simulink model "analyze"  (R2014a)
settings: Solver=FixedStepDiscrete  StartTime=0.0  StopTime=1  FixedStep=0.02  RelTol=1e-3
InitFcn:
  | Veh_Par_wxt
values from neighbouring files (symbols this model uses):
  ag_thr = 0.4*g    (= 3.924)    [Veh_Par_wxt.m]
  B = 2.25    [Veh_Par_wxt.m]
  bra_pre_em = 12    [Veh_Par_wxt.m]
  bra_pre_gz2 = 12/3    (= 4)    [Veh_Par_wxt.m]
  bra_pre_gz34 = 12/3    (= 4)    [Veh_Par_wxt.m]
  bra_pre_yd = 12/2    (= 6)    [Veh_Par_wxt.m]
  brakepre_dem_data = [0 1 2 3 4 5 6 7 8 9 10 11 12]    [Veh_Par_wxt.m]
  brakeTrq_dem_data = [0 218.198 436.396 654.594 872.792 1090.99 1309.188 1527.386 1745.584 1963.782 2181.98 2400.178 2618.376]    [Veh_Par_wxt.m]
  bratrq_max = 4*2618.376    (= 10473.504)    [Veh_Par_wxt.m]
  eff_tran = 0.75    [Veh_Par_wxt.m]
  G = Mass*g    (= 36297)    [Veh_Par_wxt.m]
  kd1 = 1    [Veh_Par_wxt.m]
  kd2 = 1    [Veh_Par_wxt.m]
  kd3 = 1    [Veh_Par_wxt.m]
  ki1 = 1    [Veh_Par_wxt.m]
  ki2 = 1    [Veh_Par_wxt.m]
  ki3 = 1    [Veh_Par_wxt.m]
  kp1 = 1    [Veh_Par_wxt.m]
  kp2 = 1    [Veh_Par_wxt.m]
  kp3 = 1    [Veh_Par_wxt.m]
  L = 3.12    [Veh_Par_wxt.m]
  premax = 12    [Veh_Par_wxt.m]
  Radius = 0.20    (= 0.2)    [Veh_Par_wxt.m]
  s_opt_yi_add = 0.05    [Veh_Par_wxt.m]
  s_opt_zhuan_add = 0.05    [Veh_Par_wxt.m]
  spd_map_mot = [0 100 200 300 360 400 500 600 700 800 900]*tras_ratio    [Veh_Par_wxt.m]
  spdmax = 900*tras_ratio    (= 5580)    [Veh_Par_wxt.m]
  speed_thr_park = 5/3.6/Radius*30/pi    (= 66.3145596216)    [Veh_Par_wxt.m]
  tras_ratio = 6.2    [Veh_Par_wxt.m]
  trq_map_mot = [1200 1200 1200 1200 1200 1080 864 720 617 540 480]/tras_ratio    [Veh_Par_wxt.m]
  trqmax = 80    [Veh_Par_wxt.m]
  v_thr1_b = 5    [Veh_Par_wxt.m]
  v_thr2_b = 20    [Veh_Par_wxt.m]
  v_thr_park = 5    [Veh_Par_wxt.m]
undefined symbols (not defined in the file or in its folder): DiscIntNeverNeededParam
libraries: simulink x231, ec5744lib x19
(part 3 of 16)

== system analyze/OutputSignalProcess/VCU_MCU2 ==
  M3Enable_in : Inport
  M3Mode_in : Inport  Port=2
  M3Drive_in : Inport  Port=3
  M3TorqueSet_in : Inport  Port=4
  M3SpeedLimit_in : Inport  Port=5
  M4Enable_in : Inport  Port=6
  M4Mode_in : Inport  Port=7
  M4Drive_in : Inport  Port=8
  M4TorqueSet_in : Inport  Port=9
  M4SpeedLimit_in : Inport  Port=10
  MCU2HeartBeat_in : Inport  Port=11
  Conv{1..8} (8 alike) : DataTypeConversion
  M3Drive : Subsystem
  M3Enable : Subsystem
  M3Mode : Subsystem
  M3SpeedLimit : Subsystem
  M3TorqueSet : Subsystem
  M4Drive : Subsystem
  M4Enable : Subsystem
  M4Mode : Subsystem
  M4SpeedLimit : Subsystem
  M4TorqueSet : Subsystem
  MCU2HeartBeat : Subsystem
  VCU_MCU2_DLC : Constant  Value=8  OutDataTypeStr=uint8
  VCU_MCU2_DLC_Out : Terminator
  VCU_MCU2_ID : Constant  Value=2348937218  OutDataTypeStr=single
  VCU_MCU2_ID_Out : Terminator
  VCU_MCU2_mux : Mux  Inputs=8
  or{1..8} (8 alike) : simulink/Logic and Bit Operations/Bitwise Operator  logicop=OR  UseBitMask=off  NumInputPorts=11  BitMask=bin2dec('11011001')  BitMaskRealWorld=Stored Integer
  output : Outport
  wires:
  VCU_MCU2_mux/1 -> output/1
  MCU2HeartBeat/1(output1) -> or1/1
  MCU2HeartBeat/2(output2) -> or2/1
  MCU2HeartBeat/3(output3) -> or3/1
  MCU2HeartBeat/4(output4) -> or4/1
  MCU2HeartBeat/5(output5) -> or5/1
  MCU2HeartBeat/6(output6) -> or6/1
  MCU2HeartBeat/7(output7) -> or7/1
  MCU2HeartBeat/8(output8) -> or8/1
  M4TorqueSet/1(output1) -> or1/2
  M4TorqueSet/2(output2) -> or2/2
  M4TorqueSet/3(output3) -> or3/2
  M4TorqueSet/4(output4) -> or4/2
  M4TorqueSet/5(output5) -> or5/2
  M4TorqueSet/6(output6) -> or6/2
  M4TorqueSet/7(output7) -> or7/2
  M4TorqueSet/8(output8) -> or8/2
  M4SpeedLimit/1(output1) -> or1/3
  M4SpeedLimit/2(output2) -> or2/3
  M4SpeedLimit/3(output3) -> or3/3
  M4SpeedLimit/4(output4) -> or4/3
  M4SpeedLimit/5(output5) -> or5/3
  M4SpeedLimit/6(output6) -> or6/3
  M4SpeedLimit/7(output7) -> or7/3
  M4SpeedLimit/8(output8) -> or8/3
  M4Mode/1(output1) -> or1/4
  M4Mode/2(output2) -> or2/4
  M4Mode/3(output3) -> or3/4
  M4Mode/4(output4) -> or4/4
  M4Mode/5(output5) -> or5/4
  M4Mode/6(output6) -> or6/4
  M4Mode/7(output7) -> or7/4
  M4Mode/8(output8) -> or8/4
  M4Enable/1(output1) -> or1/5
  M4Enable/2(output2) -> or2/5
  M4Enable/3(output3) -> or3/5
  M4Enable/4(output4) -> or4/5
  M4Enable/5(output5) -> or5/5
  M4Enable/6(output6) -> or6/5
  M4Enable/7(output7) -> or7/5
  M4Enable/8(output8) -> or8/5
  M4Drive/1(output1) -> or1/6
  M4Drive/2(output2) -> or2/6
  M4Drive/3(output3) -> or3/6
  M4Drive/4(output4) -> or4/6
  M4Drive/5(output5) -> or5/6
  M4Drive/6(output6) -> or6/6
  M4Drive/7(output7) -> or7/6
  M4Drive/8(output8) -> or8/6
  M3TorqueSet/1(output1) -> or1/7
  M3TorqueSet/2(output2) -> or2/7
  M3TorqueSet/3(output3) -> or3/7
  M3TorqueSet/4(output4) -> or4/7
  M3TorqueSet/5(output5) -> or5/7
  M3TorqueSet/6(output6) -> or6/7
  M3TorqueSet/7(output7) -> or7/7
  M3TorqueSet/8(output8) -> or8/7
  M3SpeedLimit/1(output1) -> or1/8
  M3SpeedLimit/2(output2) -> or2/8
  M3SpeedLimit/3(output3) -> or3/8
  M3SpeedLimit/4(output4) -> or4/8
  M3SpeedLimit/5(output5) -> or5/8
  M3SpeedLimit/6(output6) -> or6/8
  M3SpeedLimit/7(output7) -> or7/8
  M3SpeedLimit/8(output8) -> or8/8
  M3Mode/1(output1) -> or1/9
  M3Mode/2(output2) -> or2/9
  M3Mode/3(output3) -> or3/9
  M3Mode/4(output4) -> or4/9
  M3Mode/5(output5) -> or5/9
  M3Mode/6(output6) -> or6/9
  M3Mode/7(output7) -> or7/9
  M3Mode/8(output8) -> or8/9
  M3Enable/1(output1) -> or1/10
  M3Enable/2(output2) -> or2/10
  M3Enable/3(output3) -> or3/10
  M3Enable/4(output4) -> or4/10
  M3Enable/5(output5) -> or5/10
  M3Enable/6(output6) -> or6/10
  M3Enable/7(output7) -> or7/10
  M3Enable/8(output8) -> or8/10
  M3Drive/1(output1) -> or1/11
  M3Drive/2(output2) -> or2/11
  M3Drive/3(output3) -> or3/11
  M3Drive/4(output4) -> or4/11
  M3Drive/5(output5) -> or5/11
  M3Drive/6(output6) -> or6/11
  M3Drive/7(output7) -> or7/11
  M3Drive/8(output8) -> or8/11
  or1/1 -> Conv1/1
  Conv1/1 -> VCU_MCU2_mux/1
  or2/1 -> Conv2/1
  Conv2/1 -> VCU_MCU2_mux/2
  or3/1 -> Conv3/1
  Conv3/1 -> VCU_MCU2_mux/3
  or4/1 -> Conv4/1
  Conv4/1 -> VCU_MCU2_mux/4
  or5/1 -> Conv5/1
  Conv5/1 -> VCU_MCU2_mux/5
  or6/1 -> Conv6/1
  Conv6/1 -> VCU_MCU2_mux/6
  or7/1 -> Conv7/1
  Conv7/1 -> VCU_MCU2_mux/7
  or8/1 -> Conv8/1
  Conv8/1 -> VCU_MCU2_mux/8
  VCU_MCU2_ID/1 -> VCU_MCU2_ID_Out/1
  VCU_MCU2_DLC/1 -> VCU_MCU2_DLC_Out/1
  MCU2HeartBeat_in/1 -> MCU2HeartBeat/1(MCU2HeartBeat)
  M4TorqueSet_in/1 -> M4TorqueSet/1(M4TorqueSet)
  M4SpeedLimit_in/1 -> M4SpeedLimit/1(M4SpeedLimit)
  M4Mode_in/1 -> M4Mode/1(M4Mode)
  M4Enable_in/1 -> M4Enable/1(M4Enable)
  M4Drive_in/1 -> M4Drive/1(M4Drive)
  M3TorqueSet_in/1 -> M3TorqueSet/1(M3TorqueSet)
  M3SpeedLimit_in/1 -> M3SpeedLimit/1(M3SpeedLimit)
  M3Mode_in/1 -> M3Mode/1(M3Mode)
  M3Enable_in/1 -> M3Enable/1(M3Enable)
  M3Drive_in/1 -> M3Drive/1(M3Drive)

== matlab function analyze/MainControl/mode_control/forward/forward/Drive/驱动防滑控制TCS/转向TCS/右转/前后轮均滑转/HeartBeat1 ==
  data: life_pre input; life output
function life = fcn(life_pre)
%#codegen
life=life_pre+1;
if life>15
    life=0;
end
end

== matlab function analyze/MainControl/mode_control/forward/forward/Drive/驱动防滑控制TCS/转向TCS/右转/无滑转/HeartBeat1 ==
  data: life_pre input; life output
function life = fcn(life_pre)
%#codegen
life=life_pre+1;
if life>15
    life=0;
end
end

== matlab function analyze/MainControl/mode_control/forward/forward/Brake/MATLAB Function ==
  data: guzhang_lf input; gz_total output; guzhang_lr input; guzhang_rf input; guzhang_rr input
function gz_total = fcn(guzhang_lf,guzhang_lr,guzhang_rf,guzhang_rr)
%#codegen
if guzhang_lf==0 && guzhang_lr==0 && guzhang_rf==0 && guzhang_rr==0
    gz_total=0;
else
    gz_total=1;
end
end

== matlab function analyze/MainControl/mode_control/forward/forward/Brake/MATLAB Function1 ==
  data: syi_act_lf input; flagyi_lf output; s_opt_yi input; s_opt_yi_add input; flagyi_lf_pre input
function flagyi_lf = fcn(syi_act_lf,s_opt_yi,s_opt_yi_add,flagyi_lf_pre)
%#codegen
if syi_act_lf>s_opt_yi+s_opt_yi_add
    flagyi_lf=1;
elseif syi_act_lf<s_opt_yi
    flagyi_lf = 0;
else
    flagyi_lf=flagyi_lf_pre;
end
end

== matlab function analyze/MainControl/mode_control/forward/forward/Brake/MATLAB Function3 ==
  data: syi_act_rf input; flagyi_rf output; s_opt_yi input; s_opt_yi_add input; flagyi_rf_pre input
function flagyi_rf = fcn(syi_act_rf,s_opt_yi,s_opt_yi_add,flagyi_rf_pre)
%#codegen
if syi_act_rf>s_opt_yi+s_opt_yi_add
    flagyi_rf=1;
elseif syi_act_rf<s_opt_yi
    flagyi_rf = 0;
else
    flagyi_rf=flagyi_rf_pre;
end
end
